simulink model "Motor"  (R2021a)
settings: Solver=ode4  StartTime=0.0  StopTime=0.3  FixedStep=1e-4  RelTol=1e-3
settings Model: Creator=andim  LastModifiedBy=samu

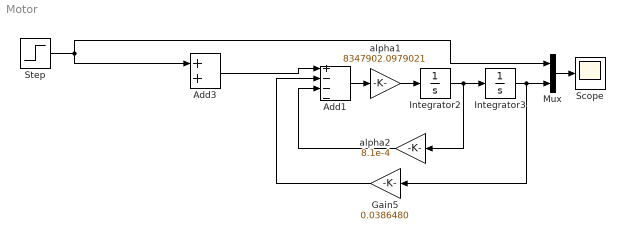
== system Motor ==
  Add1 : Sum  Inputs=+---
  Add3 : Sum
  Gain5 : Gain  Gain=0.0386480
  Integrator2 : Integrator
  Integrator3 : Integrator
  Mux : Mux  Inputs=2
  Scope : Scope
  Step : Step  Time=0.1  After=24  SampleTime=0
  alpha1 : Gain  Gain=8347902.0979021
  alpha2 : Gain  Gain=8.1e-4
  wires:
  Add1/1 -> alpha1/1
  alpha1/1 -> Integrator2/1
  Mux/1 -> Scope/1
  alpha2/1 -> Add1/3
  Gain5/1 -> Add1/2
  Integrator2/1 -> alpha2/1, Integrator3/1
  Integrator3/1 -> Gain5/1, Mux/2
  Step/1 -> Add3/1, Mux/1
  Add3/1 -> Add1/1
